simulink model "Roll_Control"  (R2022a)
settings: Solver=FixedStepAuto  StartTime=0.0  StopTime=inf  RelTol=1e-3
undefined symbols (not defined in the file): actuator, command, control, param1, param2, target_system, timestamp
libraries: ros2lib x15
settings Model: DataDictionary=Px4CmdData.sldd  Creator=30258  LastModifiedBy=30258
settings OptimizationCC: EnhancedBackFolding=on  PassReuseOutputArgsAs=Individual arguments  ZeroExternalMemoryAtStartup=off  ZeroInternalMemoryAtStartup=off  MaxStackSize=64  OptimizeBlockOrder=speed  DifferentSizesBufferReuse=on  OptimizationCustomize=off  EfficientTunableParamExpr=on
settings DebuggingCC: ParameterTunabilityLossMsg=error
settings HardwareCC: ProdBitPerLong=64  ProdLongLongMode=on  ProdHWDeviceType=Intel->x86-64 (Linux 64)
settings SFSimCC: MATLABDynamicMemAlloc=off
settings RTWCC: SystemTargetFile=ert.tlc  HardwareBoard=Robot Operating System 2 (ROS 2)  TLCOptions="-aInlineSetEventsForThisBaseRateFcn=TLC_FALSE -aSuppressMultiTaskScheduler=TLC_FALSE  -aRateBasedStepFcn=0"  TemplateMakefile=ert_default_tmf  Toolchain=Colcon Tools  TargetLang=C++
settings CodeAppCC: ForceParamTrailComments=on  IgnoreCustomStorageClasses=off  OperatorAnnotations=on  SimulinkDataObjDesc=on  SFDataObjDesc=on  InsertBlockDesc=on
settings ERTTargetCC: CodeInterfacePackaging=C++ class  ExtModeStaticAlloc=on  RootIOFormat=Structure reference

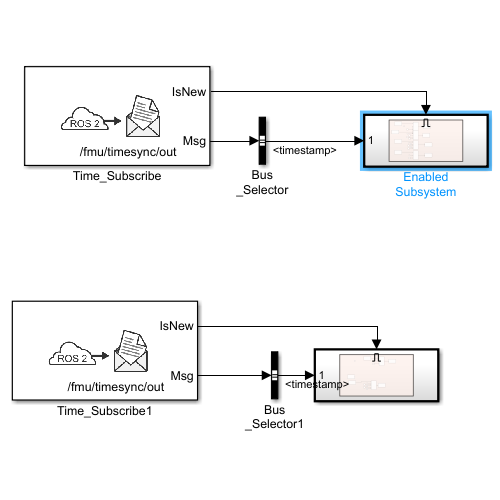
[thumbnail: Simulink's stored preview of the top-level diagram]
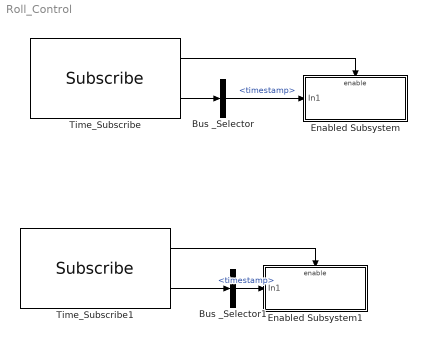
== system Roll_Control ==
  Bus _Selector : BusSelector  OutputSignals=timestamp
  Bus _Selector1 : BusSelector  OutputSignals=timestamp
  Enabled Subsystem : Subsystem  TreatAsAtomicUnit=on
  Enabled Subsystem1 : Subsystem  TreatAsAtomicUnit=on
  Time_Subscribe : ros2lib/Subscribe  topicSource=Specify your own  topic=/fmu/timesync/out  messageType=px4_msgs/Timesync  sampleTime=-1  QOSHistory=Keep last  QOSDepth=1  QOSReliability=Reliable  QOSDurability=Volatile
      settings: SourceProductBaseCode=RR
  Time_Subscribe1 : ros2lib/Subscribe  topicSource=Specify your own  topic=/fmu/timesync/out  messageType=px4_msgs/Timesync  sampleTime=-1  QOSHistory=Keep last  QOSDepth=1  QOSReliability=Reliable  QOSDurability=Volatile
      settings: SourceProductBaseCode=RR
  wires:
  Time_Subscribe/1 -> Enabled Subsystem/Enable
  Time_Subscribe/2 -> Bus _Selector/1
  Bus _Selector/1 -> Enabled Subsystem/1(In1)  "<timestamp>"
  Time_Subscribe1/2 -> Bus _Selector1/1
  Time_Subscribe1/1 -> Enabled Subsystem1/Enable
  Bus _Selector1/1 -> Enabled Subsystem1/1(In1)  "<timestamp>"

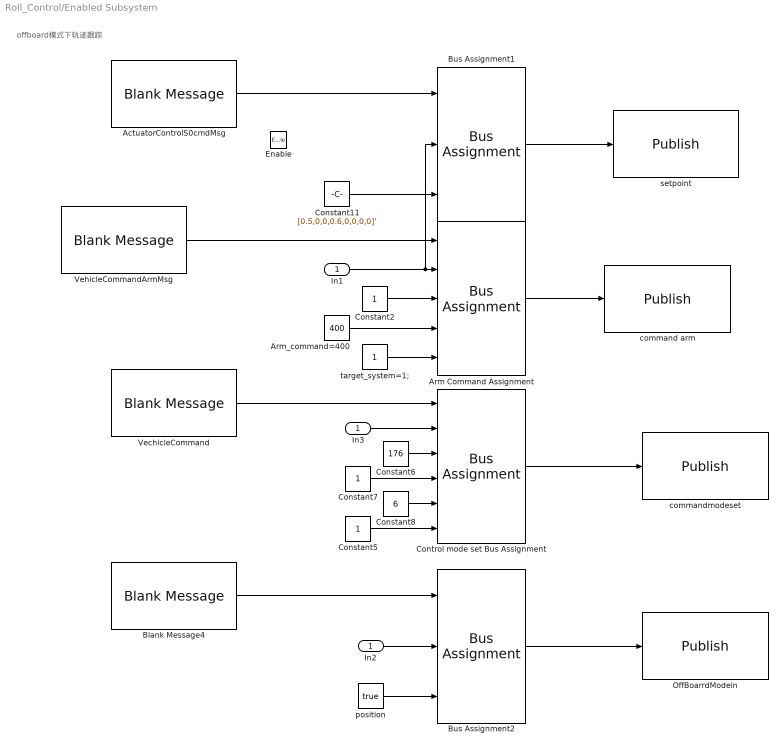
== system Roll_Control/Enabled Subsystem ==
  note: offboard模式下轨迹跟踪
  In1 : Inport
  Enable : EnablePort
  ActuatorControlS0cmdMsg : ros2lib/Blank Message  messageClass=Message  entityType=px4_msgs/ActuatorControls0  messageType=px4_msgs/ActuatorControls0  SampleTime=0.01
      settings: SourceProductBaseCode=RR
  Arm Command Assignment : BusAssignment  AssignedSignals=timestamp,param1,command,target_system
  Arm_command=400 : Constant  Value=400  OutDataTypeStr=uint32
  Blank Message4 : ros2lib/Blank Message  messageClass=Message  entityType=px4_msgs/OffboardControlMode  messageType=px4_msgs/OffboardControlMode  SampleTime=0.01
      settings: SourceProductBaseCode=RR
  Bus Assignment1 : BusAssignment  AssignedSignals=timestamp,control
  Bus Assignment2 : BusAssignment  AssignedSignals=timestamp,actuator
  Constant11 : Constant  Value=[0.5,0,0,0.6,0,0,0,0]'  VectorParams1D=off  OutDataTypeStr=single
  Constant2 : Constant  OutDataTypeStr=single
  Constant5 : Constant  OutDataTypeStr=uint8
  Constant6 : Constant  Value=176  VectorParams1D=off  OutDataTypeStr=uint32
  Constant7 : Constant  OutDataTypeStr=single
  Constant8 : Constant  Value=6  OutDataTypeStr=single
  Control mode set Bus Assignment : BusAssignment  AssignedSignals=timestamp,command,param1,param2,target_system
  In2 : InportShadow
  In3 : InportShadow
  OffBoarrdModein : ros2lib/Publish  topicSource=Specify your own  topic=/fmu/offboard_control_mode/in  messageType=px4_msgs/OffboardControlMode  QOSHistory=Keep last  QOSDepth=1  QOSReliability=Reliable  QOSDurability=Volatile
      settings: SourceProductBaseCode=RR
  VechicleCommand : ros2lib/Blank Message  messageClass=Message  entityType=px4_msgs/VehicleCommand  messageType=px4_msgs/VehicleCommand  SampleTime=0.01
      settings: SourceProductBaseCode=RR
  VehicleCommandArmMsg : ros2lib/Blank Message  messageClass=Message  entityType=px4_msgs/VehicleCommand  messageType=px4_msgs/VehicleCommand  SampleTime=0.01
      settings: SourceProductBaseCode=RR
  command arm : ros2lib/Publish  topicSource=Select from ROS network  topic=/fmu/vehicle_command/in  messageType=px4_msgs/VehicleCommand  QOSHistory=Keep last  QOSDepth=1  QOSReliability=Reliable  QOSDurability=Volatile
      settings: SourceProductBaseCode=RR
  commandmodeset : ros2lib/Publish  topicSource=Select from ROS network  topic=/fmu/vehicle_command/in  messageType=px4_msgs/VehicleCommand  QOSHistory=Keep last  QOSDepth=1  QOSReliability=Reliable  QOSDurability=Volatile
      settings: SourceProductBaseCode=RR
  position : Constant  Value=true  OutDataTypeStr=boolean
  setpoint : ros2lib/Publish  topicSource=Select from ROS network  topic=/fmu/actuator_controls0/in  messageType=px4_msgs/ActuatorControls0  QOSHistory=Keep last  QOSDepth=1  QOSReliability=Reliable  QOSDurability=Volatile
      settings: SourceProductBaseCode=RR
  target_system=1; : Constant  OutDataTypeStr=uint8
  wires:
  VehicleCommandArmMsg/1 -> Arm Command Assignment/1
  Arm_command=400/1 -> Arm Command Assignment/4
  In1/1 -> Bus Assignment1/2, Arm Command Assignment/2
  target_system=1;/1 -> Arm Command Assignment/5
  Constant2/1 -> Arm Command Assignment/3
  Arm Command Assignment/1 -> command arm/1
  Bus Assignment1/1 -> setpoint/1
  ActuatorControlS0cmdMsg/1 -> Bus Assignment1/1
  Blank Message4/1 -> Bus Assignment2/1
  Bus Assignment2/1 -> OffBoarrdModein/1
  In2/1 -> Bus Assignment2/2
  position/1 -> Bus Assignment2/3
  Control mode set Bus Assignment/1 -> commandmodeset/1
  VechicleCommand/1 -> Control mode set Bus Assignment/1
  Constant5/1 -> Control mode set Bus Assignment/6
  Constant8/1 -> Control mode set Bus Assignment/5
  In3/1 -> Control mode set Bus Assignment/2
  Constant6/1 -> Control mode set Bus Assignment/3
  Constant7/1 -> Control mode set Bus Assignment/4
  Constant11/1 -> Bus Assignment1/3

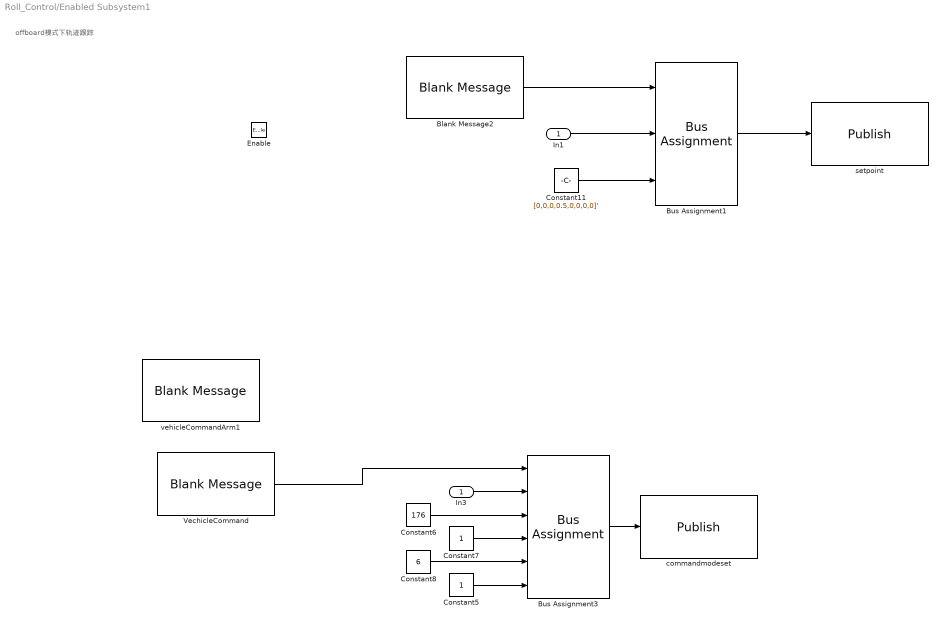
== system Roll_Control/Enabled Subsystem1 ==
  note: offboard模式下轨迹跟踪
  In1 : Inport
  Enable : EnablePort
  Blank Message2 : ros2lib/Blank Message  messageClass=Message  entityType=px4_msgs/ActuatorControls0  messageType=px4_msgs/ActuatorControls0  SampleTime=0.01
      settings: SourceProductBaseCode=RR
  Bus Assignment1 : BusAssignment  AssignedSignals=timestamp,control
  Bus Assignment3 : BusAssignment  AssignedSignals=timestamp,command,param1,param2,target_system
  Constant11 : Constant  Value=[0,0,0,0.5,0,0,0,0]'  VectorParams1D=off  OutDataTypeStr=single  SampleTime=0.02
  Constant5 : Constant  OutDataTypeStr=uint8
  Constant6 : Constant  Value=176  VectorParams1D=off  OutDataTypeStr=uint32
  Constant7 : Constant  OutDataTypeStr=single
  Constant8 : Constant  Value=6  OutDataTypeStr=single
  In3 : InportShadow
  VechicleCommand : ros2lib/Blank Message  messageClass=Message  entityType=px4_msgs/VehicleCommand  messageType=px4_msgs/VehicleCommand  SampleTime=0.01
      settings: SourceProductBaseCode=RR
  commandmodeset : ros2lib/Publish  topicSource=Select from ROS network  topic=/fmu/vehicle_command/in  messageType=px4_msgs/VehicleCommand  QOSHistory=Keep last  QOSDepth=1  QOSReliability=Reliable  QOSDurability=Volatile
      settings: SourceProductBaseCode=RR
  setpoint : ros2lib/Publish  topicSource=Select from ROS network  topic=/fmu/actuator_controls0/in  messageType=px4_msgs/ActuatorControls0  QOSHistory=Keep last  QOSDepth=1  QOSReliability=Reliable  QOSDurability=Volatile
      settings: SourceProductBaseCode=RR
  vehicleCommandArm1 : ros2lib/Blank Message  messageClass=Message  entityType=px4_msgs/VehicleAttitudeGroundtruth  messageType=px4_msgs/VehicleAttitudeGroundtruth  SampleTime=0.01
      settings: SourceProductBaseCode=RR
  wires:
  In1/1 -> Bus Assignment1/2
  Bus Assignment1/1 -> setpoint/1
  Blank Message2/1 -> Bus Assignment1/1
  Bus Assignment3/1 -> commandmodeset/1
  VechicleCommand/1 -> Bus Assignment3/1
  Constant5/1 -> Bus Assignment3/6
  Constant8/1 -> Bus Assignment3/5
  In3/1 -> Bus Assignment3/2
  Constant6/1 -> Bus Assignment3/3
  Constant7/1 -> Bus Assignment3/4
  Constant11/1 -> Bus Assignment1/3
